simulink model "Experiment_2_cs"  (Simulink 8.4)
settings: Solver=ode5  SolverMode=SingleTasking  StartTime=0.0  StopTime=inf  FixedStep=1/100  RelTol=1e-3
PreLoadFcn:
  | mbxruntime.callbacks.PreLoadFcn(bdroot);
PostLoadFcn:
  | mbxruntime.callbacks.PostLoadFcn(bdroot);
InitFcn:
  | mbxruntime.callbacks.InitFcn(bdroot);
StartFcn:
  | mbxruntime.callbacks.StartFcn(bdroot);
StopFcn:
  | mbxruntime.callbacks.StopFcn(bdroot);
undefined symbols (not defined in the file or in its folder): dfreq, gray, InitImageOutputDir, Rec, SDTV, strel, warningInitialVelocity, x0
libraries: simulink x43, PreScanSimulinkLibrary x19, visiontextngfix x15, simulink_extras x11, visionconversions x3, PreScanUsefulBlocks x3, visionsinks x2, visionstatistics x1, visionmorphops x1, visionanalysis x1
(part 2 of 8)

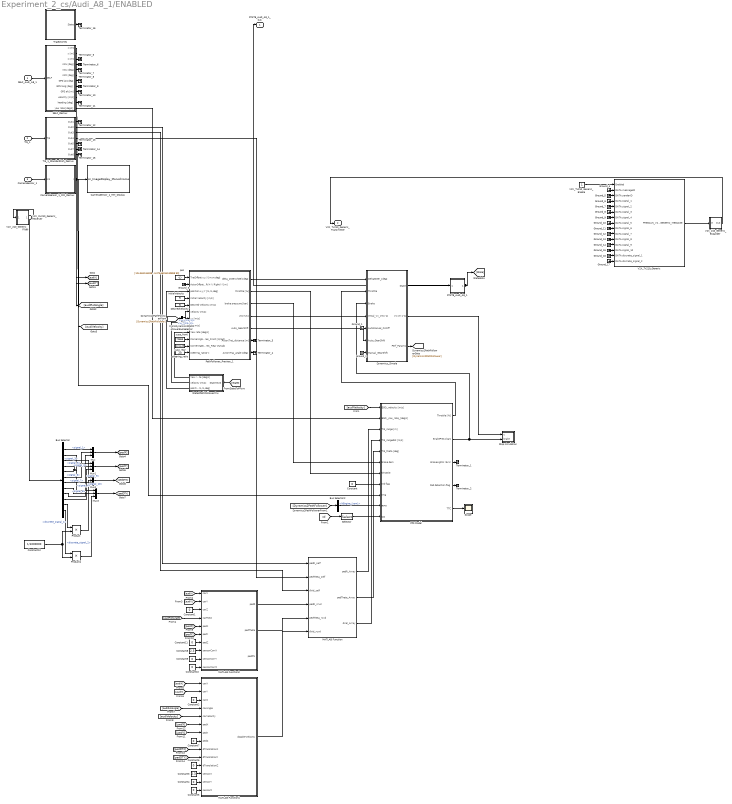
== system Experiment_2_cs/Audi_A8_1/ENABLED ==
  SELF_Audi_A8_1 : Inport  Tag=inport/SelfPort  OutDataTypeStr=Bus: PRESCAN_SELFSENSORDATA  PortDimensions=1  SampleTime=1/100  BusOutputAsStruct=on
  TIS_1 : Inport  Tag=inport/TIS  Port=2  OutDataTypeStr=Bus: PRESCAN_SCANNERSENSOR_MESSAGE  PortDimensions=3  SampleTime=1/50  BusOutputAsStruct=on
  CameraSensor_1 : Inport  Tag=inport/Camera/CameraSensor  Port=3  OutDataTypeStr=uint8  SampleTime=1/50  BusOutputAsStruct=on
  V2X_Rx210_Generic_Receiver : Inport  Tag=inport/plugin/sfun_V2X_Generic_Receiver  Port=4  BusOutputAsStruct=on
  Bus Selector : BusSelector  OutputSignals=DATA.signal_1,DATA.signal_2,DATA.signal_3,DATA.signal_4,DATA.signal_5,DATA.signal_6,DATA.signal_7,DATA.signal_8,DATA.signal_9,DATA.signal_10,DATA.discrete_signal_1,DATA.discrete_signal_2
  Bus Selector2 : BusSelector  OutputSignals=NEngine_[rpm]
  CameraSensor_1_MM_Demux : Subsystem  Tag=demux/Camera/Monochrome  mask{SensorName=CameraSensor_1, hres=500, vres=375}
      mask prompts: SensorName "Sensor Name"; hres "Horizontal Resolution"; vres "Vertical Resolution"
      mask Help: eval('openHelp(457)')
      mask Display:
      | fprintf('MONO CAMERA:\n Monochrome\n %s \n %d x %d px',SensorName,hres,vres)
      | port_label('output',1,'I')
  CameraSensor_1_MM_Display : M-S-Function  Tag=CameraSensor_Monochrome_Display  InitFcn=InitImageOutputDir(gcb);  FunctionName=fcn_ImageDisplay_Monochrome  Parameters=SensorName EnableDisplay EnablePosition DisplayPosition FigureHandle SaveResults BitmapFormat TempOutputDir CameraType DataType  mask(PreScan Monochrome Display Block){SensorName=CameraSensor_1, EnableDisplay=on, EnablePosition=off, DisplayPosition=[10 10 500 375], FigureHandle=10901, SaveResults=off, Format=PNG, TempOutputDir=0, CameraType=Mono, DataType=uint8}
      mask prompts: SensorName "User Specified: Title of Display"; EnableDisplay "Active"; EnablePosition "Set Display window position"; DisplayPosition "Display window position [xpos ypos width height]"; FigureHandle "Unique handle"; SaveResults "Save results"; TempOutputDir "OutputDir"; CameraType "Camera Type"; DataType "Image Data Type"
      mask help: This block displays the Monochrome output of a PreScan camera sensor.
      mask init:
      | if EnableDisplay
      |     EnableString='';
      |     EnableColor='gray';
      | else
      |     EnableString='INACTIVE';
      |     EnableColor='red';
      | end
      | switch Format
      |     case 1
      |         BitmapFormat = 'png';
      |     case 2
      |         BitmapFormat = 'bmp';
      |     case 3
      |         BitmapFormat = 'jpg';
      | end
      | if CameraType==1
      |     CameraTypeName='MONO';
      |     PortNumber=0;
      | else
      |     CameraTypeName='STEREO';
      |     PortNumber=1;
      | end
      settings: CopyFcn=CopyFcnDisplay  DeleteFcn=PreScanBlockDeleteFcn;  ModelCloseFcn=fcn_ImageDisplay_ModelCloseFcn
      mask Help: eval('openHelp(457)')
      mask Callback EnablePosition:
      | MV=get_param(gcb,'MaskVisibilities');
      | if strcmp(get_param(gcb,'EnablePosition'),'on')
      |     MV{4}='on';
      | else
      |     MV{4}='off';
      | end
      | set_param(gcb,'MaskVisibilities',MV);
      | clear MV;
      mask TypeOptions Format: PNG | BMP | JPG
      mask TypeOptions CameraType: Mono | Stereo
      mask TypeOptions DataType: uint8 | single
      mask Display:
      | color(EnableColor);
      | fprintf('%s\n DISPLAY:\n Monochrome\n %s',EnableString,SensorName)
      | port_label('input',1,'I')
      | port_label('input',PortNumber+1,'I')
  Constant{,1..2,4..7,9..11} (10 alike) : Constant  Value=0
  Constant12 : Constant  Value=1/1000000
  Constant3 : Constant  Value=2.3
  Constant8 : Constant  Value=2.3
  DesiredVelocity : Constant  Tag=DesiredVelocity  Value=9
  Dynamics_Simple : Subsystem  Tag=Simple_Vehicle_Dynamics  mask(PreScan Block: Simple Dynamics){Migrate=on, TimeStep=1/100, ComputationMode=Continuous_Time}
      mask prompts: Migrate "Migrate. During migration this block will be replaced by a newer one."; TimeStep "Auto assigned: Time Step [s]"; ComputationMode "Computation mode:"
      mask help:
      | The Simple Dynamics Model is selected in the GUI to simulate vehicle dynamics behavior.
      |
      | The Simple Dynamics Model is completely open to the user. The parameters of this model can be set in the Simple Dynamics dialog in the GUI.
      |
      | For more information, please click Help.
      mask init:
      | p = SimpleDyn_pars;
      settings: DeleteFcn=PreScanBlockDeleteFcn;
      mask Help: eval('openHelp(220)')
      mask Display:
      | image(imread('SimpleDyn.png'))
      | port_label('input', 1, '{\delta}_S_t_ _e_e_r [deg]','texmode','on')
      | port_label('input', 2, 'Throttle [%]')
      | port_label('input', 3, 'Brake Pres [bar]')
      | port_label('input', 4, 'V_0 [ms-1]','texmode','on')
      | port_label('input', 5, 'Auto=[0]/Manual=[1]')
      | port_label('input', 6, 'Auto_GearShift')
      | port_label('input', 7, 'Manual_GearShift')
      | port_label('output', 1, 'State')
      | port_label('output', 2, 'Vx [ms-1]')
      | port_label('output', 3, 'Perf Params')
  FromDynamics2PathFollowerBusSelector : BusSelector  OutputSignals=vx_[ms-1],vy_[ms-1]
  Ground_{1..17} (17 alike) : Ground
  InitialVelocity : Constant  Tag=InitialVelocity  Value=9
  MATLAB Function : MATLAB Function  TreatAsAtomicUnit=on
  MATLAB Function1 : MATLAB Function  TreatAsAtomicUnit=on
  MATLAB Function2 : MATLAB Function  TreatAsAtomicUnit=on
  Mux{,1..3} (4 alike) : Mux  Inputs=3
  PPS Model : Subsystem  mask(PPS Model){MaxSpeed=70, MaxBrakePressure=150, BrakeDelay=100, LaneWidth=3.5, TISMaxRange=40, TISMaxTheta=60, TISfreq=25, TISdet=32, Camfreq=50, Mainfreq=100, DisplaySwitch=on, DisplayFreq=25, RadarSwitch=on, RadarFreq=25}
      mask prompts: MaxSpeed "Vehicle cut-off speed [km/h]"; MaxBrakePressure "Maximum value of braking pressure available [bar]"; BrakeDelay "Braking system delay [ms]"; LaneWidth "Lane width [m]"; TISMaxRange "TIS maximum range [m]"; TISMaxTheta "TIS maximum theta [deg]"; TISfreq "TIS frequency [Hz]"; TISdet "Max. number of Radar detected objects [-]"; Camfreq "Camera frequency [Hz]"; Mainfreq "Compilation sheet frequency [Hz]"; DisplaySwitch "Show EGO parameters visualization"; DisplayFreq "EGO parameters visualization frequency [Hz]"; RadarSwitch "Show radar visualization"; RadarFreq "Radar frequency [Hz]"
      mask help: PreScan Experiment and Pedestrian Protection System parameters
      mask Help: eval('openHelp(8130)')
      mask Callback DisplaySwitch:
      | en = get_param(gcb,'MaskEnables');
      | switch get_param(gcb, 'DisplaySwitch')
      |     case 'off'
      |         en{12} = 'off';
      |     case 'on'
      |         en{12} = 'on';
      | end
      | set_param(gcb,'MaskEnables',en);
      mask Callback RadarSwitch:
      | en = get_param(gcb,'MaskEnables');
      | switch get_param(gcb, 'RadarSwitch')
      |     case 'off'
      |         en{14} = 'off';
      |     case 'on'
      |         en{14} = 'on';
      | end
      | set_param(gcb,'MaskEnables',en);
  PathFollower_Preview_1 : Subsystem  Tag=PathFollower_Preview  mask(PreScan Block: Path Follower with Preview){Migrate=on, FileName='Trajectory_2.mat', mass=1820, Jzz=3746, length_a=2.94 - 1.77, length_l=2.94, Angle_Max_SteeringWheel=500, PreviewTime=1, DelayTime=0.1, LowSpeedLimit=20, MaxSteeringRate=1200, CSSampleTime=1/100, PFIntegrationFrequency=100}
      mask prompts: Migrate "Migrate. During migration this block will be replaced by a newer one."; FileName "Trajectory Name"; mass "Mass vehicle total [kg]"; Jzz "Inertia vehicle around yaw axis [kg m2]"; length_a "Distance between COG and front axle [m]"; length_l "Length of wheelbase [m]"; Angle_Max_SteeringWheel "Maximum steering wheel angle [deg]"; PreviewTime "Preview time [s]"; DelayTime "Delay time [s]"; LowSpeedLimit "Low-speed limit [km/h]"; MaxSteeringRate "Maximum steering wheel angle rate [deg/s]"; CSSampleTime "Compilation Sheet sample time [s]"; PFIntegrationFrequency "Lateral controller frequency [Hz]"
      mask help:
      | The Path Follower Model is selected in the GUI to simulate driver behavior.
      |
      | For more information, please click Help.
      mask init:
      | load(['trajectories/',eval(FileName)])
      | traject=trajectory';
      | 
      | Traj_x=traject(:,2);
      | Traj_y=traject(:,3);
      | Traj_t=traject(2,1);
      | Traj_v=sqrt(traject(:,8).^2+traject(:,9).^2+traject(:,10).^2);
      | 
      | RefreshCounter = (1/CSSampleTime) / (PFIntegrationFrequency); %Compilation sheet frequency/path follower frequency
      | 
      | blockPath = gcb;
      | 
      | clear traject;
      mask Help: eval('openHelp(233)')
  Product : Product
  Product1 : Product
  SELF_Demux : Subsystem  Tag=demux/SelfPort  mask(PreScan Demux Block:){}
      mask help:
      | The SELF port shows (state) information of the actor itself. The outputs are position in the experiment's axis system and the GPS coordinates, and the object's absolute velocity and compass heading.
      |
      | For more information, please click Help.
      settings: DeleteFcn=PreScanBlockDeleteFcn;
      mask Help: eval('openHelp(462)')
      mask Display:
      | port_label('output',1,'x [m]')
      | port_label('output',2,'y [m]')
      | port_label('output',3,'z [m]','texmode','on')
      | port_label('output',4,'Rotx [deg]','texmode','on')
      | port_label('output',5,'Roty [deg]','texmode','on')
      | port_label('output',6,'Rotz [deg]','texmode','on')
      | port_label('output',7,'GPS lat [deg]','texmode','on')
      | port_label('output',8,'GPS long [deg]','texmode','on')
      | port_label('output',9,'GPS alt [m]','texmode','on')
      | port_label('output',10,'Velocity [m/s]')
      | port_label('output',11,'Heading [deg]')
      | port_label('output',12,'Yaw rate [deg/s]')
  STATE_Audi_A8_1 : Subsystem  Tag=mux/StatePort  Priority=0  LoadFcn=load PrescanStateActuatorData  mask(PreScan Sink Block: State){x0=124.56113433837891, y0=125.07546234130859, z0=0.55, Roll0=0, Pitch0=0, Yaw0=90, TimeStep=1/100}
      mask prompts: x0 "Ini x-position VEHICLE wrt GLOBAL axis system [m]"; y0 "Ini y-position VEHICLE wrt GLOBAL axis system [m]"; z0 "Ini z-position VEHICLE wrt GLOBAL axis system [m]"; Roll0 "Ini roll-angle BODY wrt VEHICLE axis system [deg]"; Pitch0 "Ini pitch-angle BODY wrt VEHICLE axis system [deg]"; Yaw0 "Ini yaw-angle VEHICLE wrt GLOBAL axis system [deg]"; TimeStep "Auto-Assigned: Upload Period [s]"
      mask help:
      | The Actor State contains a vector signal of size (9x1), containing the following signals:
      |
      | -  Position                  (x,y,z)                                     [m]
      | -  Velocity                  (vx,vy,vz)                               [m/s]
      | -  Angles                    (Roll, Pitch, Yaw)                   [rad]
      |
      | The Actor state is defined in the global axis system.
      | The state is superponed on the Initial position defined in the GUI.
      |
      | For more information, please click Help.
      settings: DeleteFcn=PreScanBlockDeleteFcn;
      mask Help: eval('openHelp(222)')
      mask Display: image(imread('State.png'))
  Scope : Scope
  Selector : Selector  InputPortWidth=5
  State2PathFollowerCnv : Subsystem  Tag=State2PFConnection/cnv
  Stop simulation : Subsystem
  TIS_1_StandardCoh_Demux : Subsystem  Tag=demux/TIS/StandardCoh  TreatAsAtomicUnit=on  mask(PreScan Demux Block: TIS){MAXMESSAGES=3}
      mask prompts: MAXMESSAGES "Number of Objects"
      mask Help: eval('openHelp(449)')
      mask Display:
      | port_label('input',1,'TIS')
      | port_label('output',1,'Beam ID [-]')
      | port_label('output',2,'Range [m]')
      | port_label('output',3,'DopplerVelocity [m/s]')
      | port_label('output',4,'{\theta} [deg]','texmode','on')
      | port_label('output',5,'{\phi} [deg]','texmode','on')
      | port_label('output',6,'Target ID [-]','texmode','on')
      | port_label('output',7,'TIS Data','texmode','on')
  Terminator_{1..16} (16 alike) : Terminator
  Trajectories : Subsystem  Tag=Trajectories  mask(PreScan Source Block: Trajectories){}
      mask help:
      | The Trajectory block contains the trajectories defined in the PreScan Experiment Editor. The output of the trajectory block is the (vehicle) State.
      |
      | For more information, please click Help.
      settings: DeleteFcn=PreScanBlockDeleteFcn;
      mask Help: eval('openHelp(312)')
      mask Display: image(imread('Trajectory.png'));
  V2X_210_Generic_Expander : Subsystem  LoadFcn=addpath .\V2XPlugin; V2Xbusses;
  V2X_210_Generic_Filter : Subsystem
      mask Display: disp('[1]');
  V2X_Tx210_Generic : Subsystem
  V2X_Tx210_Generic_Enable : Constant  OutDataTypeStr=Inherit: Inherit via back propagation
  pos : Constant  Tag=pos  Value=[124.56113433837891 125.07546234130859 90]
  steering_ratio : Constant  Tag=steering_ratio  Value=20
  susp_front : Constant  Tag=susp_front  Value=72653
  susp_rear : Constant  Tag=susp_rear  Value=121449
  STATE_Audi_A8_1_bus : Outport  Tag=outport/StatePort  OutDataTypeStr=Bus: PRESCAN_STATEACTUATORDATA  PortDimensions=1  SampleTime=1/100
  V2X_Tx210_Generic_Transmitter : Outport  Tag=outport/plugin/sfun_V2X_Generic_Transmitter  Port=2
  wires:
  CameraSensor_1_MM_Demux/1(I) -> PPS Model/9(img), CameraSensor_1_MM_Display/1
  Dynamics_Simple/2(Vx [m s-1]) -> Stop simulation/1(V)
  SELF_Demux/1(x [m]) -> [audiX]
  SELF_Demux/2(y [m]) -> [audiY]
  SELF_Demux/6(rotz [deg]) -> [audiRotAngle]
  SELF_Demux/10(velocity [m/s]) -> [audiVelocity]
  TIS_1_StandardCoh_Demux/2(Out2) -> MATLAB Function/1(pedR_self)
  V2X_210_Generic_Filter/1(Filter_Out) -> Bus Selector/1
  MATLAB Function2/3(pedPhi) -> ?
  [audiX] -> MATLAB Function2/1(carX)
  [audiY] -> MATLAB Function2/2(carY)
  Constant1/1 -> MATLAB Function2/3(carZ)
  [audiRotAngle] -> MATLAB Function2/4(carRotZ)
  [audiX] -> MATLAB Function1/1(carX)
  [audiY] -> MATLAB Function1/2(carY)
  Constant2/1 -> MATLAB Function1/3(carZ)
  [audiRotAngle] -> MATLAB Function1/4(carAngle)
  [audiVelocity] -> MATLAB Function1/5(carVelocity)
  Constant3/1 -> MATLAB Function1/12(sensorX)
  Constant4/1 -> MATLAB Function1/13(sensorY)
  Constant5/1 -> MATLAB Function1/14(sensorZ)
  Constant6/1 -> MATLAB Function1/11(dTranslationZ)
  Constant7/1 -> MATLAB Function1/8(pedZ)
  Constant8/1 -> MATLAB Function2/8(sensorCorrX)
  Constant9/1 -> MATLAB Function2/9(sensorCorrY)
  Constant10/1 -> MATLAB Function2/10(sensorCorrZ)
  Constant11/1 -> MATLAB Function2/7(pedZ)
  [pedX] -> MATLAB Function2/5(pedX)
  [pedY] -> MATLAB Function2/6(pedY)
  [pedX] -> MATLAB Function1/6(pedX)
  [pedY] -> MATLAB Function1/7(pedY)
  [pedDTX] -> MATLAB Function1/9(dTranslationX)
  [pedDTY] -> MATLAB Function1/10(dTranslationY)
  Bus Selector2/1 -> PPS Model/10(RPM)  "<NEngine_[rpm]>"
  Selector/1 -> PPS Model/11(CD)
  [cd] -> Selector/1
  Constant/1 -> PPS Model/8(ind flag)
  PPS Model/5(TTC) -> Scope/1
  PPS Model/2(BrakePres [bar]) -> Dynamics_Simple/3(Brake), Stop simulation/2(brake)
  [audiVelocity] -> PPS Model/1(EGO_velocity [m/s])
  SELF_Demux/12(yaw rate [deg/s]) -> PPS Model/2(EGO_yaw_rate_[deg/s])
  PathFollower_Preview_1/2(throttle [%]) -> PPS Model/7(throttle)
  PathFollower_Preview_1/3(brake pressure [bar]) -> PPS Model/6(brake dem)
  PPS Model/1(Throttle [%]) -> Dynamics_Simple/2(Throttle)
  TIS_1_StandardCoh_Demux/3(Out3) -> MATLAB Function/3(dVel_self)
  TIS_1_StandardCoh_Demux/4(Out4) -> MATLAB Function/2(pedTheta_self)
  [Dynamics2PathFollower] -> Bus Selector2/1
  Bus Selector/1 -> Mux/1  "<signal_1>"
  Bus Selector/5 -> Mux/2  "<signal_5>"
  Mux/1 -> [pedX]
  Bus Selector/2 -> Mux1/1  "<signal_2>"
  Bus Selector/6 -> Mux1/2  "<signal_6>"
  Mux1/1 -> [pedY]
  Bus Selector/3 -> Mux2/1  "<signal_3>"
  Bus Selector/7 -> Mux2/2  "<signal_7>"
  Mux2/1 -> [pedDTX]
  Mux3/1 -> [pedDTY]
  Bus Selector/4 -> Mux3/1  "<signal_4>"
  Bus Selector/8 -> Mux3/2  "<signal_8>"
  Bus Selector/9 -> Mux/3  "<signal_9>"
  Bus Selector/10 -> Mux1/3  "<signal_10>"
  Constant12/1 -> Product/2, Product1/2
  Bus Selector/11 -> Product/1  "<discrete_signal_1>"
  Product/1 -> Mux2/3
  Bus Selector/12 -> Product1/1  "<discrete_signal_2>"
  Product1/1 -> Mux3/3
  MATLAB Function/1(pedR_Array) -> PPS Model/3(TIS_range [m])
  MATLAB Function/2(pedTheta_Array) -> PPS Model/5(TIS_theta [deg])
  MATLAB Function/3(dVel_Array) -> PPS Model/4(TIS_rangedot [m/s])
  MATLAB Function2/1(pedR) -> MATLAB Function/4(pedR_rcvd)
  MATLAB Function2/2(pedTheta) -> MATLAB Function/5(pedTheta_rcvd)
  MATLAB Function1/1(dopplerVelocity) -> MATLAB Function/6(dVel_rcvd)
  STATE_Audi_A8_1/1(StateBus) -> STATE_Audi_A8_1_bus/1, [State]
  SELF_Audi_A8_1/1 -> SELF_Demux/1(SELF)
  TIS_1/1 -> TIS_1_StandardCoh_Demux/1(TIS)
  CameraSensor_1/1 -> CameraSensor_1_MM_Demux/1(In1)
  pos/1 -> PathFollower_Preview_1/1(TrajOffset x,y,Y [m,m,deg])
  susp_front/1 -> PathFollower_Preview_1/10(CorneringStiffness_Tyres_Front [N/rad])
  susp_rear/1 -> PathFollower_Preview_1/11(CorneringStiffness_Tyres_Rear [N/rad])
  steering_ratio/1 -> PathFollower_Preview_1/12(steering_ratio[-])
  InitialVelocity/1 -> PathFollower_Preview_1/4(Initial Velocity [m/s])
  DesiredVelocity/1 -> PathFollower_Preview_1/5(Desired Velocity [m/s])
  [State] -> State2PathFollowerCnv/1(State BUS)
  State2PathFollowerCnv/1(Yaw rate [deg/s]) -> PathFollower_Preview_1/9(Yaw rate [deg/s])
  State2PathFollowerCnv/2(velocity [m/s]) -> PathFollower_Preview_1/6(velocity [m/s])
  State2PathFollowerCnv/3(position x,y,Y [m,m,deg]) -> PathFollower_Preview_1/3(position x,y,Y [m,m,deg])
  PathFollower_Preview_1/1(delta_steerwheel [deg]) -> Dynamics_Simple/1(DeltaSteer_[deg])
  PathFollower_Preview_1/4(v0 [m/s]) -> Dynamics_Simple/4(Initial_Vx_[ms-1])
  PathFollower_Preview_1/5(Auto_GearShift) -> Dynamics_Simple/6(Auto_GearShift)
  Dynamics_Simple/3(Perf_Params) -> [Dynamics2PathFollower]
  FromDynamics2PathFollowerBusSelector/1 -> PathFollower_Preview_1/7(vx [m/s])  "<vx_[ms-1]>"
  FromDynamics2PathFollowerBusSelector/2 -> PathFollower_Preview_1/8(vy [m/s])  "<vy_[ms-1]>"
  [Dynamics2PathFollower] -> FromDynamics2PathFollowerBusSelector/1
  Dynamics_Simple/1(State) -> STATE_Audi_A8_1/1(State)
  V2X_Tx210_Generic_Enable/1 -> V2X_Tx210_Generic/1(Enabled)
  V2X_Tx210_Generic/1(PRESCAN_V2X_USER_GENERIC_MESSAGE) -> V2X_210_Generic_Expander/1(In)
  V2X_210_Generic_Expander/1(Out) -> V2X_Tx210_Generic_Transmitter/1
  V2X_Rx210_Generic_Receiver/1 -> V2X_210_Generic_Filter/1(Filter_In)
  Ground_1/1 -> Dynamics_Simple/5(AutoManual_OnOff)
  Ground_2/1 -> Dynamics_Simple/7(Manual_GearShift)
  PPS Model/3(BrakeLights (3x1)) -> Terminator_1/1
  PPS Model/4(Ped detection flag) -> Terminator_2/1
  Ground_3/1 -> PathFollower_Preview_1/2(ActorOffset_Left(+) / Right(-) [m])
  PathFollower_Preview_1/6(Actor/Traj_distance [m]) -> Terminator_3/1
  PathFollower_Preview_1/7(Actor/Traj_angle [deg]) -> Terminator_4/1
  SELF_Demux/3(z [m]) -> Terminator_5/1
  SELF_Demux/4(rotx [deg]) -> Terminator_6/1
  SELF_Demux/5(roty [deg]) -> Terminator_7/1
  SELF_Demux/7(GPS lat [deg]) -> Terminator_8/1
  SELF_Demux/8(GPS long [deg]) -> Terminator_9/1
  SELF_Demux/9(GPS alt [m]) -> Terminator_10/1
  SELF_Demux/11(heading [deg]) -> Terminator_11/1
  TIS_1_StandardCoh_Demux/1(Out1) -> Terminator_12/1
  TIS_1_StandardCoh_Demux/5(Out5) -> Terminator_13/1
  TIS_1_StandardCoh_Demux/6(Out7) -> Terminator_14/1
  TIS_1_StandardCoh_Demux/7(Out6) -> Terminator_15/1
  Trajectories/1(State) -> Terminator_16/1
  Ground_4/1 -> V2X_Tx210_Generic/2(DATA.messageID)
  Ground_5/1 -> V2X_Tx210_Generic/3(DATA.senderID)
  Ground_6/1 -> V2X_Tx210_Generic/4(DATA.signal_1)
  Ground_7/1 -> V2X_Tx210_Generic/5(DATA.signal_2)
  Ground_8/1 -> V2X_Tx210_Generic/6(DATA.signal_3)
  Ground_9/1 -> V2X_Tx210_Generic/7(DATA.signal_4)
  Ground_10/1 -> V2X_Tx210_Generic/8(DATA.signal_5)
  Ground_11/1 -> V2X_Tx210_Generic/9(DATA.signal_6)
  Ground_12/1 -> V2X_Tx210_Generic/10(DATA.signal_7)
  Ground_13/1 -> V2X_Tx210_Generic/11(DATA.signal_8)
  Ground_14/1 -> V2X_Tx210_Generic/12(DATA.signal_9)
  Ground_15/1 -> V2X_Tx210_Generic/13(DATA.signal_10)
  Ground_16/1 -> V2X_Tx210_Generic/14(DATA.discrete_signal_1)
  Ground_17/1 -> V2X_Tx210_Generic/15(DATA.discrete_signal_2)

== system Experiment_2_cs/BMW_Z3_1/DISABLED ==
  SELF_BMW_Z3_1 : Inport  Tag=inport/SelfPort  OutDataTypeStr=Bus: PRESCAN_SELFSENSORDATA  PortDimensions=1  SampleTime=1/100  BusOutputAsStruct=on
  TIS_2 : Inport  Tag=inport/TIS  Port=2  OutDataTypeStr=Bus: PRESCAN_SCANNERSENSOR_MESSAGE  PortDimensions=3  SampleTime=1/50  BusOutputAsStruct=on
  V2X_Rx211_Generic_Receiver : Inport  Tag=inport/plugin/sfun_V2X_Generic_Receiver  Port=3  BusOutputAsStruct=on
  GND1 : Subsystem
  GND2 : Ground
  TRM1 : Terminator
  TRM2 : Terminator
  TRM3 : Terminator
  STATE_BMW_Z3_1_bus : Outport  Tag=outport/StatePort  OutDataTypeStr=Bus: PRESCAN_STATEACTUATORDATA  PortDimensions=1  SampleTime=1/100
  V2X_Tx211_Generic_Transmitter : Outport  Tag=outport/plugin/sfun_V2X_Generic_Transmitter  Port=2
  wires:
  SELF_BMW_Z3_1/1 -> TRM1/1
  TIS_2/1 -> TRM2/1
  V2X_Rx211_Generic_Receiver/1 -> TRM3/1
  GND1/1(bus) -> STATE_BMW_Z3_1_bus/1
  GND2/1 -> V2X_Tx211_Generic_Transmitter/1

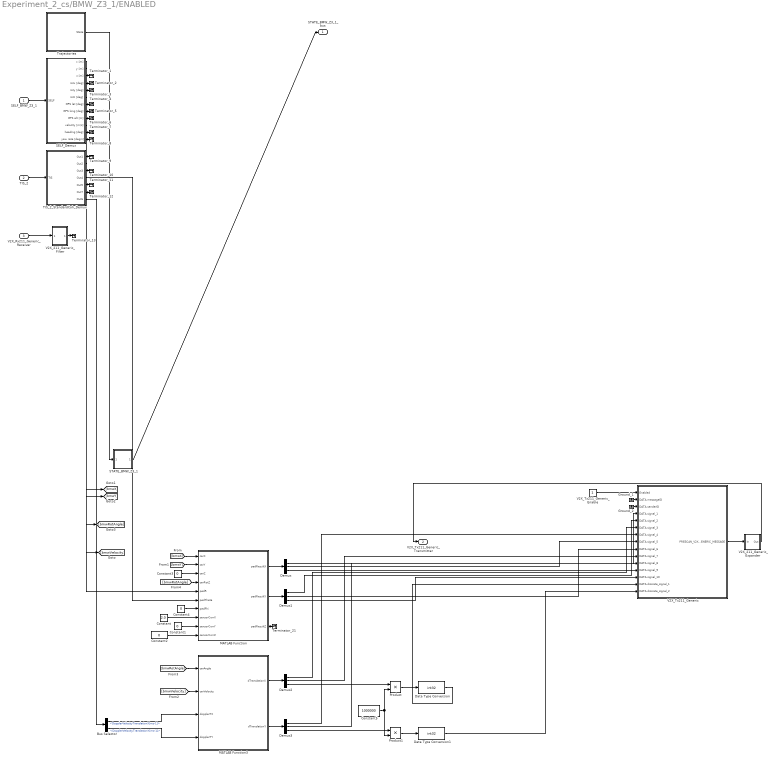
== system Experiment_2_cs/BMW_Z3_1/ENABLED ==
  SELF_BMW_Z3_1 : Inport  Tag=inport/SelfPort  OutDataTypeStr=Bus: PRESCAN_SELFSENSORDATA  PortDimensions=1  SampleTime=1/100  BusOutputAsStruct=on
  TIS_2 : Inport  Tag=inport/TIS  Port=2  OutDataTypeStr=Bus: PRESCAN_SCANNERSENSOR_MESSAGE  PortDimensions=3  SampleTime=1/50  BusOutputAsStruct=on
  V2X_Rx211_Generic_Receiver : Inport  Tag=inport/plugin/sfun_V2X_Generic_Receiver  Port=3  BusOutputAsStruct=on
  Bus Selector : BusSelector  OutputSignals=DopplerVelocityTranslationX[ms-1],DopplerVelocityTranslationY[ms-1]
  Constant : Constant  Value=2.0
  Constant{1..4} (4 alike) : Constant  Value=0
  Constant5 : Constant  Value=1000000
  Data Type Conversion : DataTypeConversion  OutDataTypeStr=int32
  Data Type Conversion1 : DataTypeConversion  OutDataTypeStr=int32
  Demux{,1..3} (4 alike) : Demux  Outputs=3
  Ground_1 : Ground
  Ground_2 : Ground
  MATLAB Function : MATLAB Function  TreatAsAtomicUnit=on
  MATLAB Function3 : MATLAB Function  TreatAsAtomicUnit=on
  Product : Product
  Product1 : Product
  SELF_Demux : Subsystem  Tag=demux/SelfPort  mask(PreScan Demux Block:){}
      mask help:
      | The SELF port shows (state) information of the actor itself. The outputs are position in the experiment's axis system and the GPS coordinates, and the object's absolute velocity and compass heading.
      |
      | For more information, please click Help.
      settings: DeleteFcn=PreScanBlockDeleteFcn;
      mask Help: eval('openHelp(462)')
      mask Display:
      | port_label('output',1,'x [m]')
      | port_label('output',2,'y [m]')
      | port_label('output',3,'z [m]','texmode','on')
      | port_label('output',4,'Rotx [deg]','texmode','on')
      | port_label('output',5,'Roty [deg]','texmode','on')
      | port_label('output',6,'Rotz [deg]','texmode','on')
      | port_label('output',7,'GPS lat [deg]','texmode','on')
      | port_label('output',8,'GPS long [deg]','texmode','on')
      | port_label('output',9,'GPS alt [m]','texmode','on')
      | port_label('output',10,'Velocity [m/s]')
      | port_label('output',11,'Heading [deg]')
      | port_label('output',12,'Yaw rate [deg/s]')
  STATE_BMW_Z3_1 : Subsystem  Tag=mux/StatePort  Priority=0  LoadFcn=load PrescanStateActuatorData  mask(PreScan Sink Block: State){x0=49.386848449707031, y0=148.20474243164062, z0=0.4784, Roll0=0, Pitch0=0, Yaw0=7.7315318591786308E-09, TimeStep=1/100}
      mask prompts: x0 "Ini x-position VEHICLE wrt GLOBAL axis system [m]"; y0 "Ini y-position VEHICLE wrt GLOBAL axis system [m]"; z0 "Ini z-position VEHICLE wrt GLOBAL axis system [m]"; Roll0 "Ini roll-angle BODY wrt VEHICLE axis system [deg]"; Pitch0 "Ini pitch-angle BODY wrt VEHICLE axis system [deg]"; Yaw0 "Ini yaw-angle VEHICLE wrt GLOBAL axis system [deg]"; TimeStep "Auto-Assigned: Upload Period [s]"
      mask help:
      | The Actor State contains a vector signal of size (9x1), containing the following signals:
      |
      | -  Position                  (x,y,z)                                     [m]
      | -  Velocity                  (vx,vy,vz)                               [m/s]
      | -  Angles                    (Roll, Pitch, Yaw)                   [rad]
      |
      | The Actor state is defined in the global axis system.
      | The state is superponed on the Initial position defined in the GUI.
      |
      | For more information, please click Help.
      settings: DeleteFcn=PreScanBlockDeleteFcn;
      mask Help: eval('openHelp(222)')
      mask Display: image(imread('State.png'))
  TIS_2_StandardCoh_Demux : Subsystem  Tag=demux/TIS/StandardCoh  TreatAsAtomicUnit=on  mask(PreScan Demux Block: TIS){MAXMESSAGES=3}
      mask prompts: MAXMESSAGES "Number of Objects"
      mask Help: eval('openHelp(449)')
      mask Display:
      | port_label('input',1,'TIS')
      | port_label('output',1,'Beam ID [-]')
      | port_label('output',2,'Range [m]')
      | port_label('output',3,'DopplerVelocity [m/s]')
      | port_label('output',4,'{\theta} [deg]','texmode','on')
      | port_label('output',5,'{\phi} [deg]','texmode','on')
      | port_label('output',6,'Target ID [-]','texmode','on')
      | port_label('output',7,'TIS Data','texmode','on')
  Terminator_{1..13,21} (14 alike) : Terminator
  Trajectories : Subsystem  Tag=Trajectories  mask(PreScan Source Block: Trajectories){}
      mask help:
      | The Trajectory block contains the trajectories defined in the PreScan Experiment Editor. The output of the trajectory block is the (vehicle) State.
      |
      | For more information, please click Help.
      settings: DeleteFcn=PreScanBlockDeleteFcn;
      mask Help: eval('openHelp(312)')
      mask Display: image(imread('Trajectory.png'));
  V2X_211_Generic_Expander : Subsystem  LoadFcn=addpath .\V2XPlugin; V2Xbusses;
  V2X_211_Generic_Filter : Subsystem
      mask Display: disp('[1]');
  V2X_Tx211_Generic : Subsystem
  V2X_Tx211_Generic_Enable : Constant  OutDataTypeStr=Inherit: Inherit via back propagation
  STATE_BMW_Z3_1_bus : Outport  Tag=outport/StatePort  OutDataTypeStr=Bus: PRESCAN_STATEACTUATORDATA  PortDimensions=1  SampleTime=1/100
  V2X_Tx211_Generic_Transmitter : Outport  Tag=outport/plugin/sfun_V2X_Generic_Transmitter  Port=2
  wires:
  TIS_2_StandardCoh_Demux/2(Out2) -> MATLAB Function/5(pedR)
  TIS_2_StandardCoh_Demux/4(Out4) -> MATLAB Function/6(pedTheta)
  TIS_2_StandardCoh_Demux/7(Out6) -> Bus Selector/1
  Constant/1 -> MATLAB Function/8(sensorCorrX)
  Constant1/1 -> MATLAB Function/9(sensorCorrY)
  Constant2/1 -> MATLAB Function/10(sensorCorrZ)
  Constant3/1 -> MATLAB Function/3(carZ)
  Constant4/1 -> MATLAB Function/7(pedPhi)
  Bus Selector/1 -> MATLAB Function3/3(dopplerTX)  "<DopplerVelocityTranslationX[ms-1]>"
  Bus Selector/2 -> MATLAB Function3/4(dopplerTY)  "<DopplerVelocityTranslationY[ms-1]>"
  [bmwX] -> MATLAB Function/1(carX)
  [bmwY] -> MATLAB Function/2(carY)
  [bmwVelocity] -> MATLAB Function3/2(carVelocity)
  [bmwRotAngle] -> MATLAB Function3/1(carAngle)
  [bmwRotAngle] -> MATLAB Function/4(carRotZ)
  MATLAB Function/3(pedResultZ) -> Terminator_21/1
  SELF_Demux/1(x [m]) -> [bmwX]
  SELF_Demux/2(y [m]) -> [bmwY]
  SELF_Demux/6(rotz [deg]) -> [bmwRotAngle]
  SELF_Demux/10(velocity [m/s]) -> [bmwVelocity]
  MATLAB Function/1(pedResultX) -> Demux/1
  MATLAB Function/2(pedResultY) -> Demux1/1
  MATLAB Function3/1(dTranslationX) -> Demux2/1
  MATLAB Function3/2(dTranslationY) -> Demux3/1
  Demux/1 -> V2X_Tx211_Generic/4(DATA.signal_1)
  Demux1/1 -> V2X_Tx211_Generic/5(DATA.signal_2)
  Demux2/1 -> V2X_Tx211_Generic/6(DATA.signal_3)
  Demux3/1 -> V2X_Tx211_Generic/7(DATA.signal_4)
  Demux/2 -> V2X_Tx211_Generic/8(DATA.signal_5)
  Demux1/2 -> V2X_Tx211_Generic/9(DATA.signal_6)
  Demux2/2 -> V2X_Tx211_Generic/10(DATA.signal_7)
  Demux3/2 -> V2X_Tx211_Generic/11(DATA.signal_8)
  Demux/3 -> V2X_Tx211_Generic/12(DATA.signal_9)
  Demux1/3 -> V2X_Tx211_Generic/13(DATA.signal_10)
  Demux2/3 -> Product/1
  Demux3/3 -> Product1/1
  Constant5/1 -> Product/2, Product1/2
  Product/1 -> Data Type Conversion/1
  Data Type Conversion/1 -> V2X_Tx211_Generic/14(DATA.discrete_signal_1)
  Product1/1 -> Data Type Conversion1/1
  Data Type Conversion1/1 -> V2X_Tx211_Generic/15(DATA.discrete_signal_2)
  STATE_BMW_Z3_1/1(StateBus) -> STATE_BMW_Z3_1_bus/1
  SELF_BMW_Z3_1/1 -> SELF_Demux/1(SELF)
  TIS_2/1 -> TIS_2_StandardCoh_Demux/1(TIS)
  Trajectories/1(State) -> STATE_BMW_Z3_1/1(State)
  V2X_Tx211_Generic_Enable/1 -> V2X_Tx211_Generic/1(Enabled)
  V2X_Tx211_Generic/1(PRESCAN_V2X_USER_GENERIC_MESSAGE) -> V2X_211_Generic_Expander/1(In)
  V2X_211_Generic_Expander/1(Out) -> V2X_Tx211_Generic_Transmitter/1
  V2X_Rx211_Generic_Receiver/1 -> V2X_211_Generic_Filter/1(Filter_In)
  SELF_Demux/3(z [m]) -> Terminator_1/1
  SELF_Demux/4(rotx [deg]) -> Terminator_2/1
  SELF_Demux/5(roty [deg]) -> Terminator_3/1
  SELF_Demux/7(GPS lat [deg]) -> Terminator_4/1
  SELF_Demux/8(GPS long [deg]) -> Terminator_5/1
  SELF_Demux/9(GPS alt [m]) -> Terminator_6/1
  SELF_Demux/11(heading [deg]) -> Terminator_7/1
  SELF_Demux/12(yaw rate [deg/s]) -> Terminator_8/1
  TIS_2_StandardCoh_Demux/1(Out1) -> Terminator_9/1
  TIS_2_StandardCoh_Demux/3(Out3) -> Terminator_10/1
  TIS_2_StandardCoh_Demux/5(Out5) -> Terminator_11/1
  TIS_2_StandardCoh_Demux/6(Out7) -> Terminator_12/1
  V2X_211_Generic_Filter/1(Filter_Out) -> Terminator_13/1
  Ground_1/1 -> V2X_Tx211_Generic/2(DATA.messageID)
  Ground_2/1 -> V2X_Tx211_Generic/3(DATA.senderID)

== system Experiment_2_cs/CameraSensor_1/DISABLED ==
  GND1 : Ground
  CameraSensor_1 : Outport  Tag=outport/Camera/CameraSensor  OutDataTypeStr=uint8  SampleTime=1/50
  wires:
  GND1/1 -> CameraSensor_1/1

== system Experiment_2_cs/CameraSensor_1/ENABLED ==
  Sensor : S-Function  FunctionName=sfun_Camera  Parameters=sensorID, dataWidth, dataHeight, channelsPerImage, numberOfImages, timestep  EnableBusSupport=off  mask(PreScan Source Block: Camera Sensor){sensorID=207, dataWidth=375, dataHeight=500, channelsPerImage=1, numberOfImages=1, timestep=1/50}
      mask prompts: sensorID "Sensor ID"; dataWidth "Data width"; dataHeight "Data Height"; channelsPerImage "Channels per image"; numberOfImages "Number of images"; timestep "MATLAB timestep:"
      mask help: The Camera Sensor provides a color or monochrome image.
      mask Help: eval('openHelp(457)')
      mask Display: image(imread('CameraSensor.png'))
  CameraSensor_1 : Outport  Tag=outport/Camera/CameraSensor  OutDataTypeStr=uint8  SampleTime=1/50
  wires:
  Sensor/1 -> CameraSensor_1/1

== system Experiment_2_cs/CollisionDetection/DISABLED ==
  GND1 : Subsystem
  CollisionDetection : Outport  Tag=outport/CollisionDetection  OutDataTypeStr=Bus: PRESCAN_COLLISIONDETECTION_MESSAGE  PortDimensions=5  SampleTime=1/100
  wires:
  GND1/1(bus) -> CollisionDetection/1

== system Experiment_2_cs/CollisionDetection/ENABLED ==
  Sensor : S-Function  FunctionName=sfun_CollisionDetection  Parameters=detectableCollisions, timestep  EnableBusSupport=off  mask(PreScan Source Block: CollisionDetection){detectableCollisions=5, timestep=1/100}
      mask prompts: detectableCollisions "Max detectable collisions:"; timestep "MATLAB timestep:"
      mask help: Collision Detection can be used to detect collisions between PreScan components. For Collision Detection the actual component shape is taken into account, so it is not a bounding box approach.
      mask Help: eval('openHelp(811)')
      mask Display: image(imread('crash.jpg'))
  CollisionDetection : Outport  Tag=outport/CollisionDetection  OutDataTypeStr=Bus: PRESCAN_COLLISIONDETECTION_MESSAGE  PortDimensions=5  SampleTime=1/100
  wires:
  Sensor/1 -> CollisionDetection/1

== system Experiment_2_cs/Male_RegularAni_1/DISABLED ==
  SELF_Male_RegularAni_1 : Inport  Tag=inport/SelfPort  OutDataTypeStr=Bus: PRESCAN_SELFSENSORDATA  PortDimensions=1  SampleTime=1/100  BusOutputAsStruct=on
  GND1 : Subsystem
  GND2 : Subsystem
  TRM1 : Terminator
  STATE_Male_RegularAni_1_bus : Outport  Tag=outport/StatePort  OutDataTypeStr=Bus: PRESCAN_STATEACTUATORDATA  PortDimensions=1  SampleTime=1/100
  ANIM_Male_RegularAni_1 : Outport  Tag=outport/AnimationOutport  Port=2  OutDataTypeStr=Bus: PRESCAN_ANIMACTUATORDATA  PortDimensions=1  SampleTime=1/100
  wires:
  SELF_Male_RegularAni_1/1 -> TRM1/1
  GND1/1(bus) -> STATE_Male_RegularAni_1_bus/1
  GND2/1(bus) -> ANIM_Male_RegularAni_1/1

== system Experiment_2_cs/Male_RegularAni_1/ENABLED ==
  SELF_Male_RegularAni_1 : Inport  Tag=inport/SelfPort  OutDataTypeStr=Bus: PRESCAN_SELFSENSORDATA  PortDimensions=1  SampleTime=1/100  BusOutputAsStruct=on
  Animation : Subsystem  Tag=RunningHumanAnimation  mask(Prescan Conversion Block: Running Human Animation){MWS=1.95, WalkingScale=1.0, RunningScale=1.0, TimeStep=1/100}
      mask prompts: MWS "Maximum Walking Speed [m/s], above which the animation will switch to running mode."; WalkingScale "Walking mode scaling factor to sync the animation frames to the displacement."; RunningScale "Running mode scaling factor to sync the animation frames to the displacement."; TimeStep "Auto-Assigned: Upload Period [s]"
      mask help: The Running Human Animation block converts the State signal of a human into signals to properly control the animation.
      mask Help: eval('openHelp(239)');
      mask Display: image(imread('HumanAnimated.jpg'))
  SELF_Demux : Subsystem  Tag=demux/SelfPort  mask(PreScan Demux Block:){}
      mask help:
      | The SELF port shows (state) information of the actor itself. The outputs are position in the experiment's axis system and the GPS coordinates, and the object's absolute velocity and compass heading.
      |
      | For more information, please click Help.
      settings: DeleteFcn=PreScanBlockDeleteFcn;
      mask Help: eval('openHelp(462)')
      mask Display:
      | port_label('output',1,'x [m]')
      | port_label('output',2,'y [m]')
      | port_label('output',3,'z [m]','texmode','on')
      | port_label('output',4,'Rotx [deg]','texmode','on')
      | port_label('output',5,'Roty [deg]','texmode','on')
      | port_label('output',6,'Rotz [deg]','texmode','on')
      | port_label('output',7,'GPS lat [deg]','texmode','on')
      | port_label('output',8,'GPS long [deg]','texmode','on')
      | port_label('output',9,'GPS alt [m]','texmode','on')
      | port_label('output',10,'Velocity [m/s]')
      | port_label('output',11,'Heading [deg]')
      | port_label('output',12,'Yaw rate [deg/s]')
  STATE_Male_RegularAni_1 : Subsystem  Tag=mux/StatePort  Priority=0  LoadFcn=load PrescanStateActuatorData  mask(PreScan Sink Block: State){x0=91.173126220703125, y0=141.368896484375, z0=0, Roll0=0, Pitch0=0, Yaw0=90.216752291554755, TimeStep=1/100}
      mask prompts: x0 "Ini x-position VEHICLE wrt GLOBAL axis system [m]"; y0 "Ini y-position VEHICLE wrt GLOBAL axis system [m]"; z0 "Ini z-position VEHICLE wrt GLOBAL axis system [m]"; Roll0 "Ini roll-angle BODY wrt VEHICLE axis system [deg]"; Pitch0 "Ini pitch-angle BODY wrt VEHICLE axis system [deg]"; Yaw0 "Ini yaw-angle VEHICLE wrt GLOBAL axis system [deg]"; TimeStep "Auto-Assigned: Upload Period [s]"
      mask help:
      | The Actor State contains a vector signal of size (9x1), containing the following signals:
      |
      | -  Position                  (x,y,z)                                     [m]
      | -  Velocity                  (vx,vy,vz)                               [m/s]
      | -  Angles                    (Roll, Pitch, Yaw)                   [rad]
      |
      | The Actor state is defined in the global axis system.
      | The state is superponed on the Initial position defined in the GUI.
      |
      | For more information, please click Help.
      settings: DeleteFcn=PreScanBlockDeleteFcn;
      mask Help: eval('openHelp(222)')
      mask Display: image(imread('State.png'))
  Terminator_{1..12} (12 alike) : Terminator
  Trajectories : Subsystem  Tag=Trajectories  mask(PreScan Source Block: Trajectories){}
      mask help:
      | The Trajectory block contains the trajectories defined in the PreScan Experiment Editor. The output of the trajectory block is the (vehicle) State.
      |
      | For more information, please click Help.
      settings: DeleteFcn=PreScanBlockDeleteFcn;
      mask Help: eval('openHelp(312)')
      mask Display: image(imread('Trajectory.png'));
  STATE_Male_RegularAni_1_bus : Outport  Tag=outport/StatePort  OutDataTypeStr=Bus: PRESCAN_STATEACTUATORDATA  PortDimensions=1  SampleTime=1/100
  ANIM_Male_RegularAni_1 : Outport  Tag=outport/AnimationOutport  Port=2  OutDataTypeStr=Bus: PRESCAN_ANIMACTUATORDATA  PortDimensions=1  SampleTime=1/100
  wires:
  STATE_Male_RegularAni_1/1(StateBus) -> STATE_Male_RegularAni_1_bus/1, Animation/1(In1)
  Animation/1(Out1) -> ANIM_Male_RegularAni_1/1
  SELF_Male_RegularAni_1/1 -> SELF_Demux/1(SELF)
  Trajectories/1(State) -> STATE_Male_RegularAni_1/1(State)
  SELF_Demux/1(x [m]) -> Terminator_1/1
  SELF_Demux/2(y [m]) -> Terminator_2/1
  SELF_Demux/3(z [m]) -> Terminator_3/1
  SELF_Demux/4(rotx [deg]) -> Terminator_4/1
  SELF_Demux/5(roty [deg]) -> Terminator_5/1
  SELF_Demux/6(rotz [deg]) -> Terminator_6/1
  SELF_Demux/7(GPS lat [deg]) -> Terminator_7/1
  SELF_Demux/8(GPS long [deg]) -> Terminator_8/1
  SELF_Demux/9(GPS alt [m]) -> Terminator_9/1
  SELF_Demux/10(velocity [m/s]) -> Terminator_10/1
  SELF_Demux/11(heading [deg]) -> Terminator_11/1
  SELF_Demux/12(yaw rate [deg/s]) -> Terminator_12/1

== system Experiment_2_cs/SELF_Audi_A8_1/DISABLED ==
  GND1 : Subsystem
  SELF_Audi_A8_1 : Outport  Tag=outport/SelfPort  OutDataTypeStr=Bus: PRESCAN_SELFSENSORDATA  PortDimensions=1  SampleTime=1/100
  wires:
  GND1/1(bus) -> SELF_Audi_A8_1/1

== system Experiment_2_cs/SELF_Audi_A8_1/ENABLED ==
  Sensor : S-Function  FunctionName=sfun_SelfSensor  Parameters=UniqueID, TimeStep  EnableBusSupport=off  mask(PreScan Source Block: SELF){UniqueID=109, TimeStep=1/100}
      mask prompts: UniqueID "Auto-Assigned: Unique ID"; TimeStep "Auto-Assigned: Upload Period [s]"
      mask help:
      | The SELF port shows (state) information of the actor itself. The outputs are position in the experiment's axis system and the GPS coordinates, and the object's absolute velocity and compass heading.
      |
      | For more information, please click Help.
      mask Help: eval('openHelp(462)')
      mask Display: image(imread('GPS.png'))
  SELF_Audi_A8_1 : Outport  Tag=outport/SelfPort  OutDataTypeStr=Bus: PRESCAN_SELFSENSORDATA  PortDimensions=1  SampleTime=1/100
  wires:
  Sensor/1 -> SELF_Audi_A8_1/1

== system Experiment_2_cs/SELF_BMW_Z3_1/DISABLED ==
  GND1 : Subsystem
  SELF_BMW_Z3_1 : Outport  Tag=outport/SelfPort  OutDataTypeStr=Bus: PRESCAN_SELFSENSORDATA  PortDimensions=1  SampleTime=1/100
  wires:
  GND1/1(bus) -> SELF_BMW_Z3_1/1

== system Experiment_2_cs/SELF_BMW_Z3_1/ENABLED ==
  Sensor : S-Function  FunctionName=sfun_SelfSensor  Parameters=UniqueID, TimeStep  EnableBusSupport=off  mask(PreScan Source Block: SELF){UniqueID=112, TimeStep=1/100}
      mask prompts: UniqueID "Auto-Assigned: Unique ID"; TimeStep "Auto-Assigned: Upload Period [s]"
      mask help:
      | The SELF port shows (state) information of the actor itself. The outputs are position in the experiment's axis system and the GPS coordinates, and the object's absolute velocity and compass heading.
      |
      | For more information, please click Help.
      mask Help: eval('openHelp(462)')
      mask Display: image(imread('GPS.png'))
  SELF_BMW_Z3_1 : Outport  Tag=outport/SelfPort  OutDataTypeStr=Bus: PRESCAN_SELFSENSORDATA  PortDimensions=1  SampleTime=1/100
  wires:
  Sensor/1 -> SELF_BMW_Z3_1/1

== system Experiment_2_cs/SELF_Male_RegularAni_1/DISABLED ==
  GND1 : Subsystem
  SELF_Male_RegularAni_1 : Outport  Tag=outport/SelfPort  OutDataTypeStr=Bus: PRESCAN_SELFSENSORDATA  PortDimensions=1  SampleTime=1/100
  wires:
  GND1/1(bus) -> SELF_Male_RegularAni_1/1

== system Experiment_2_cs/SELF_Male_RegularAni_1/ENABLED ==
  Sensor : S-Function  FunctionName=sfun_SelfSensor  Parameters=UniqueID, TimeStep  EnableBusSupport=off  mask(PreScan Source Block: SELF){UniqueID=116, TimeStep=1/100}
      mask prompts: UniqueID "Auto-Assigned: Unique ID"; TimeStep "Auto-Assigned: Upload Period [s]"
      mask help:
      | The SELF port shows (state) information of the actor itself. The outputs are position in the experiment's axis system and the GPS coordinates, and the object's absolute velocity and compass heading.
      |
      | For more information, please click Help.
      mask Help: eval('openHelp(462)')
      mask Display: image(imread('GPS.png'))
  SELF_Male_RegularAni_1 : Outport  Tag=outport/SelfPort  OutDataTypeStr=Bus: PRESCAN_SELFSENSORDATA  PortDimensions=1  SampleTime=1/100
  wires:
  Sensor/1 -> SELF_Male_RegularAni_1/1

== system Experiment_2_cs/STATE_Audi_A8_1_bus/DISABLED ==
  STATE_Audi_A8_1_bus : Inport  Tag=inport/StatePort  OutDataTypeStr=Bus: PRESCAN_STATEACTUATORDATA  PortDimensions=1  SampleTime=1/100  BusOutputAsStruct=on
  TRM1 : Terminator
  wires:
  STATE_Audi_A8_1_bus/1 -> TRM1/1

== system Experiment_2_cs/STATE_Audi_A8_1_bus/ENABLED ==
  STATE_Audi_A8_1_bus : Inport  Tag=inport/StatePort  OutDataTypeStr=Bus: PRESCAN_STATEACTUATORDATA  PortDimensions=1  SampleTime=1/100  BusOutputAsStruct=on
  Actuator : S-Function  FunctionName=sfun_StateActuator  Parameters=UniqueID, TimeStep  EnableBusSupport=off  mask(PreScan Sink Block: State){UniqueID=109, TimeStep=1/100}
      mask prompts: UniqueID "Auto-Assigned: Unique ID"; TimeStep "Auto-Assigned: Upload Period [s]"
      mask help:
      | The Actor State contains a vector signal of size (9x1), containing the following signals:
      |
      | -  Position    	(x,y,z)             	[m]
      | -  Velocity    	(vx,vy,vz)         	[m/s]
      | -  Angles       	(Roll, Pitch, Yaw)	[rad]
      |
      | The Actor state is defined in the global axis system.
      | The state is superponed on the Initial position defined in the GUI.
      |
      | For more information, please click Help.
      mask Help: eval('openHelp(222)')
      mask Display: image(imread('State.png'))
  wires:
  STATE_Audi_A8_1_bus/1 -> Actuator/1

== system Experiment_2_cs/STATE_BMW_Z3_1_bus/DISABLED ==
  STATE_BMW_Z3_1_bus : Inport  Tag=inport/StatePort  OutDataTypeStr=Bus: PRESCAN_STATEACTUATORDATA  PortDimensions=1  SampleTime=1/100  BusOutputAsStruct=on
  TRM1 : Terminator
  wires:
  STATE_BMW_Z3_1_bus/1 -> TRM1/1

== system Experiment_2_cs/STATE_BMW_Z3_1_bus/ENABLED ==
  STATE_BMW_Z3_1_bus : Inport  Tag=inport/StatePort  OutDataTypeStr=Bus: PRESCAN_STATEACTUATORDATA  PortDimensions=1  SampleTime=1/100  BusOutputAsStruct=on
  Actuator : S-Function  FunctionName=sfun_StateActuator  Parameters=UniqueID, TimeStep  EnableBusSupport=off  mask(PreScan Sink Block: State){UniqueID=112, TimeStep=1/100}
      mask prompts: UniqueID "Auto-Assigned: Unique ID"; TimeStep "Auto-Assigned: Upload Period [s]"
      mask help:
      | The Actor State contains a vector signal of size (9x1), containing the following signals:
      |
      | -  Position    	(x,y,z)             	[m]
      | -  Velocity    	(vx,vy,vz)         	[m/s]
      | -  Angles       	(Roll, Pitch, Yaw)	[rad]
      |
      | The Actor state is defined in the global axis system.
      | The state is superponed on the Initial position defined in the GUI.
      |
      | For more information, please click Help.
      mask Help: eval('openHelp(222)')
      mask Display: image(imread('State.png'))
  wires:
  STATE_BMW_Z3_1_bus/1 -> Actuator/1

== system Experiment_2_cs/STATE_Male_RegularAni_1_bus/DISABLED ==
  STATE_Male_RegularAni_1_bus : Inport  Tag=inport/StatePort  OutDataTypeStr=Bus: PRESCAN_STATEACTUATORDATA  PortDimensions=1  SampleTime=1/100  BusOutputAsStruct=on
  TRM1 : Terminator
  wires:
  STATE_Male_RegularAni_1_bus/1 -> TRM1/1

== system Experiment_2_cs/STATE_Male_RegularAni_1_bus/ENABLED ==
  STATE_Male_RegularAni_1_bus : Inport  Tag=inport/StatePort  OutDataTypeStr=Bus: PRESCAN_STATEACTUATORDATA  PortDimensions=1  SampleTime=1/100  BusOutputAsStruct=on
  Actuator : S-Function  FunctionName=sfun_StateActuator  Parameters=UniqueID, TimeStep  EnableBusSupport=off  mask(PreScan Sink Block: State){UniqueID=116, TimeStep=1/100}
      mask prompts: UniqueID "Auto-Assigned: Unique ID"; TimeStep "Auto-Assigned: Upload Period [s]"
      mask help:
      | The Actor State contains a vector signal of size (9x1), containing the following signals:
      |
      | -  Position    	(x,y,z)             	[m]
      | -  Velocity    	(vx,vy,vz)         	[m/s]
      | -  Angles       	(Roll, Pitch, Yaw)	[rad]
      |
      | The Actor state is defined in the global axis system.
      | The state is superponed on the Initial position defined in the GUI.
      |
      | For more information, please click Help.
      mask Help: eval('openHelp(222)')
      mask Display: image(imread('State.png'))
  wires:
  STATE_Male_RegularAni_1_bus/1 -> Actuator/1

== system Experiment_2_cs/TIS_1/DISABLED ==
  GND1 : Subsystem
  TIS_1 : Outport  Tag=outport/TIS  OutDataTypeStr=Bus: PRESCAN_SCANNERSENSOR_MESSAGE  PortDimensions=3  SampleTime=1/50
  wires:
  GND1/1(bus) -> TIS_1/1

== system Experiment_2_cs/TIS_1/ENABLED ==
  Sensor : S-Function  FunctionName=sfun_TIS  Parameters=sensorID, detectableObjects, timestep  EnableBusSupport=off  mask(PreScan Source Block: Technology Independent Sensor (TIS)){sensorID=203, detectableObjects=3, timestep=1/50}
      mask prompts: sensorID "Sensor ID"; detectableObjects "Max detectable objects:"; timestep "MATLAB timestep:"
      mask help:
      | The Technology Independent Sensor (TIS) provides a sensor with all sensor-related influence factors (like noise, drift and accuracy) without being technology specific (like radar and lidar). The TIS detects the closest point on the geometry of an object.
      |
      | For more information, please click Help.
      mask Help: eval('openHelp(449)')
      mask Display: image(imread('TIS.png'))
  TIS_1 : Outport  Tag=outport/TIS  OutDataTypeStr=Bus: PRESCAN_SCANNERSENSOR_MESSAGE  PortDimensions=3  SampleTime=1/50
  wires:
  Sensor/1 -> TIS_1/1

== system Experiment_2_cs/TIS_2/DISABLED ==
  GND1 : Subsystem
  TIS_2 : Outport  Tag=outport/TIS  OutDataTypeStr=Bus: PRESCAN_SCANNERSENSOR_MESSAGE  PortDimensions=3  SampleTime=1/50
  wires:
  GND1/1(bus) -> TIS_2/1

== system Experiment_2_cs/TIS_2/ENABLED ==
  Sensor : S-Function  FunctionName=sfun_TIS  Parameters=sensorID, detectableObjects, timestep  EnableBusSupport=off  mask(PreScan Source Block: Technology Independent Sensor (TIS)){sensorID=206, detectableObjects=3, timestep=1/50}
      mask prompts: sensorID "Sensor ID"; detectableObjects "Max detectable objects:"; timestep "MATLAB timestep:"
      mask help:
      | The Technology Independent Sensor (TIS) provides a sensor with all sensor-related influence factors (like noise, drift and accuracy) without being technology specific (like radar and lidar). The TIS detects the closest point on the geometry of an object.
      |
      | For more information, please click Help.
      mask Help: eval('openHelp(449)')
      mask Display: image(imread('TIS.png'))
  TIS_2 : Outport  Tag=outport/TIS  OutDataTypeStr=Bus: PRESCAN_SCANNERSENSOR_MESSAGE  PortDimensions=3  SampleTime=1/50
  wires:
  Sensor/1 -> TIS_2/1

== system Experiment_2_cs/V2X_Rx210_Generic_Receiver/DISABLED ==
  GND1 : Ground
  V2X_Rx210_Generic_Receiver : Outport  Tag=outport/plugin/sfun_V2X_Generic_Receiver
  wires:
  GND1/1 -> V2X_Rx210_Generic_Receiver/1

== system Experiment_2_cs/V2X_Rx210_Generic_Receiver/ENABLED ==
  Sensor : S-Function  LoadFcn=load('Generic.mat');  FunctionName=sfun_V2X_Generic_Receiver  Parameters=sensorID, parentID, maxMessages, timestep  EnableBusSupport=off  mask(V2X Generic Receiver Block){sensorID=210, parentID=109, maxMessages=1, timestep=1/100}
      mask prompts: sensorID "Receiver ID"; parentID "Parent ID"; maxMessages "Maximum number of messages"; timestep "MATLAB timestep:"
      mask help: V2X Block receiving a Generic message
      mask Display: image(imread('V2XR_grayscale.png'))
  V2X_Rx210_Generic_Receiver : Outport  Tag=outport/plugin/sfun_V2X_Generic_Receiver
  wires:
  Sensor/1 -> V2X_Rx210_Generic_Receiver/1

== system Experiment_2_cs/V2X_Rx211_Generic_Receiver/DISABLED ==
  GND1 : Ground
  V2X_Rx211_Generic_Receiver : Outport  Tag=outport/plugin/sfun_V2X_Generic_Receiver
  wires:
  GND1/1 -> V2X_Rx211_Generic_Receiver/1

== system Experiment_2_cs/V2X_Rx211_Generic_Receiver/ENABLED ==
  Sensor : S-Function  LoadFcn=load('Generic.mat');  FunctionName=sfun_V2X_Generic_Receiver  Parameters=sensorID, parentID, maxMessages, timestep  EnableBusSupport=off  mask(V2X Generic Receiver Block){sensorID=211, parentID=112, maxMessages=1, timestep=1/100}
      mask prompts: sensorID "Receiver ID"; parentID "Parent ID"; maxMessages "Maximum number of messages"; timestep "MATLAB timestep:"
      mask help: V2X Block receiving a Generic message
      mask Display: image(imread('V2XR_grayscale.png'))
  V2X_Rx211_Generic_Receiver : Outport  Tag=outport/plugin/sfun_V2X_Generic_Receiver
  wires:
  Sensor/1 -> V2X_Rx211_Generic_Receiver/1

== system Experiment_2_cs/V2X_Tx210_Generic_Transmitter/DISABLED ==
  V2X_Tx210_Generic_Transmitter : Inport  Tag=inport/plugin/sfun_V2X_Generic_Transmitter  BusOutputAsStruct=on
  TRM1 : Terminator
  wires:
  V2X_Tx210_Generic_Transmitter/1 -> TRM1/1

== system Experiment_2_cs/V2X_Tx210_Generic_Transmitter/ENABLED ==
  V2X_Tx210_Generic_Transmitter : Inport  Tag=inport/plugin/sfun_V2X_Generic_Transmitter  BusOutputAsStruct=on
  Actuator : S-Function  LoadFcn=load('Generic.mat');  FunctionName=sfun_V2X_Generic_Transmitter  Parameters=sensorID, parentID, timestep  EnableBusSupport=off  mask(V2X Generic Transmitter Block){sensorID=210, parentID=109, timestep=1/100}
      mask prompts: sensorID "Transmitter ID"; parentID "Parent ID"; timestep "MATLAB timestep:"
      mask help: V2X Block transmitting a Generic message
      mask Display: image(imread('V2XT_grayscale.png'))
  wires:
  V2X_Tx210_Generic_Transmitter/1 -> Actuator/1

== system Experiment_2_cs/V2X_Tx211_Generic_Transmitter/DISABLED ==
  V2X_Tx211_Generic_Transmitter : Inport  Tag=inport/plugin/sfun_V2X_Generic_Transmitter  BusOutputAsStruct=on
  TRM1 : Terminator
  wires:
  V2X_Tx211_Generic_Transmitter/1 -> TRM1/1
